simulink model "L3G4200D_SPI_interface"  (R2015a)
settings: Solver=FixedStepDiscrete  SolverMode=SingleTasking  StartTime=0.0  StopTime=inf  FixedStep=.001  RelTol=1e-3
model workspace (MAT data in the model file):
  message_length = Simulink.Parameter
  message_length.Value = 16
  message_length.DataType = 'uint16'
  clk_freq = Simulink.Parameter
  clk_freq.Value = 1000000
  clk_freq.DataType = 'uint32'
  cs_to_clk_edge = Simulink.Parameter
  cs_to_clk_edge.Value = 10
  cs_to_clk_edge.DataType = 'uint16'
  stall_time = Simulink.Parameter
  stall_time.Value = 4
  stall_time.DataType = 'uint16'
  Tcount_max = 20
  Tstall_max = 2000
  PAGE_0 = 32768
  PAGE_1 = 32769
  PAGE_2 = 32770
  PAGE_3 = 32771
  DEC_RATE_984a = 35864
  DEC_RATE_984b = 36096
  Z_ACCL_OUT = 9728
  PROD_ID = 32256
  CTRL_REG1_L3G = 8399
  OUT_X_L_L3G = 43008
  OUT_X_H_L3G = 43264
  OUT_Y_L_L3G = 43520
  OUT_Y_H_L3G = 43776
  OUT_Z_L_L3G = 44032
  OUT_Z_H_L3G = 44288
  read_table_L3G = [43008 43264 43520 43776 44032 44288 36608]
  WHO_AM_I_L3G = 36608
  init_cmd_L3G = 8399
undefined symbols (not defined in the file): AXI4, Lite
libraries: axiinterfacelib x8
settings Model: FPTRunName=FPA_Reference  SimulationMode=external  RecordCoverage=on  CovPath=/hdl_dut/Transmit  CovMetricSettings=r  CovHtmlReporting=off  CovReportOnPause=off  CovSFcnEnable=off  Creator=dlwalter  LastModifiedBy=dlwalter
settings OptimizationCC: BlockReduction=off  BooleanDataType=off  ConditionallyExecuteInputs=off  OptimizeModelRefInitCode=on  LifeSpan=2  MaxStackSize=64
settings DebuggingCC: AlgebraicLoopMsg=error  SaveWithParameterizedLinksMsg=none  UnderspecifiedInitializationDetection=Classic  MergeDetectMultiDrivingBlocksExec=none  SignalResolutionControl=TryResolveAllWithWarning
settings HardwareCC: ProdLargestAtomicInteger=Long  ProdLargestAtomicFloat=Double  ProdEndianess=LittleEndian  ProdHWDeviceType=ARM Compatible->ARM Cortex  TargetUnknown=on  ProdEqTarget=off
settings RTWCC: SystemTargetFile=ert.tlc  TLCOptions=-aInlineSetEventsForThisBaseRateFcn=TLC_FALSE -aSuppressMultiTaskScheduler=TLC_FALSE  TemplateMakefile=ert_default_tmf  Description=Embedded Coder  Toolchain=Xilinx Software Development Kit (SDK) 2013.4
settings CodeAppCC: IgnoreCustomStorageClasses=off
settings ERTTargetCC: GenerateSampleERTMain=off  ParMdlRefBuildCompliant=on  CompOptLevelCompliant=on  ConcurrentExecutionCompliant=on  ERTFirstTimeCompliant=on  SupportContinuousTime=off  SupportVariableSizeSignals=off  ModelStepFunctionPrototypeControlCompliant=on  CPPClassGenCompliant=on

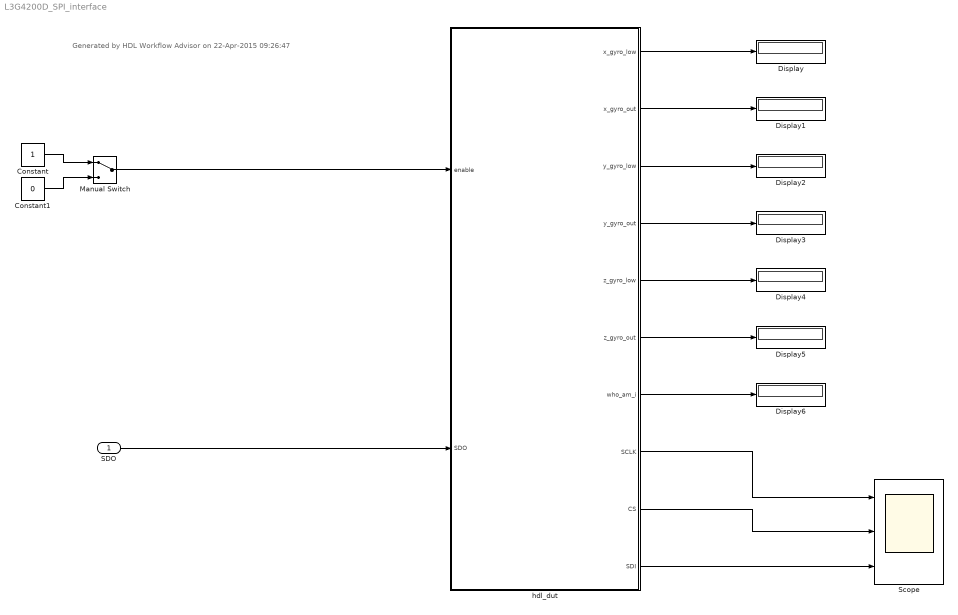
== system L3G4200D_SPI_interface ==
  note: Generated by HDL Workflow Advisor on 22-Apr-2015 09:26:47
  SDO : Inport
  Constant : Constant  OutDataTypeStr=boolean  SampleTime=-1
  Constant1 : Constant  Value=0  OutDataTypeStr=boolean  SampleTime=-1
  Display{,1..6} (7 alike) : Display
      Display6 settings: Format=octal (Stored Integer)
  Manual Switch : ManualSwitch
  Scope : Scope  NumInputPorts=3
      settings: TimeRange=3000  YMin=-5~-5~-5  YMax=5~5~5
  hdl_dut : Subsystem  TreatAsAtomicUnit=on  MinMaxOverflowLogging=MinMaxAndOverflow  mask(AXI4-Lite/AXI4 Interface){}
      mask help:
      | This is an automatically generated subsystem block.
      | This contains the AXI4-Lite/AXI4 interface which communicates with the L3G4200D_SPI_hdl_dut_ipcore IPCore generated from L3G4200D_SPI/hdl_dut subsystem.
      mask Display: disp(sprintf('Xilinx Zynq \nAXI4-Lite/AXI4 Interface'));
  wires:
  Constant1/1 -> Manual Switch/2
  Constant/1 -> Manual Switch/1
  hdl_dut/10(SDI) -> Scope/3
  hdl_dut/9(CS) -> Scope/2
  hdl_dut/8(SCLK) -> Scope/1
  hdl_dut/7(who_am_i) -> Display6/1
  hdl_dut/5(z_gyro_low) -> Display4/1
  hdl_dut/6(z_gyro_out) -> Display5/1
  hdl_dut/4(y_gyro_out) -> Display3/1
  hdl_dut/3(y_gyro_low) -> Display2/1
  hdl_dut/2(x_gyro_out) -> Display1/1
  hdl_dut/1(x_gyro_low) -> Display/1
  SDO/1 -> hdl_dut/2(SDO)
  Manual Switch/1 -> hdl_dut/1(enable)

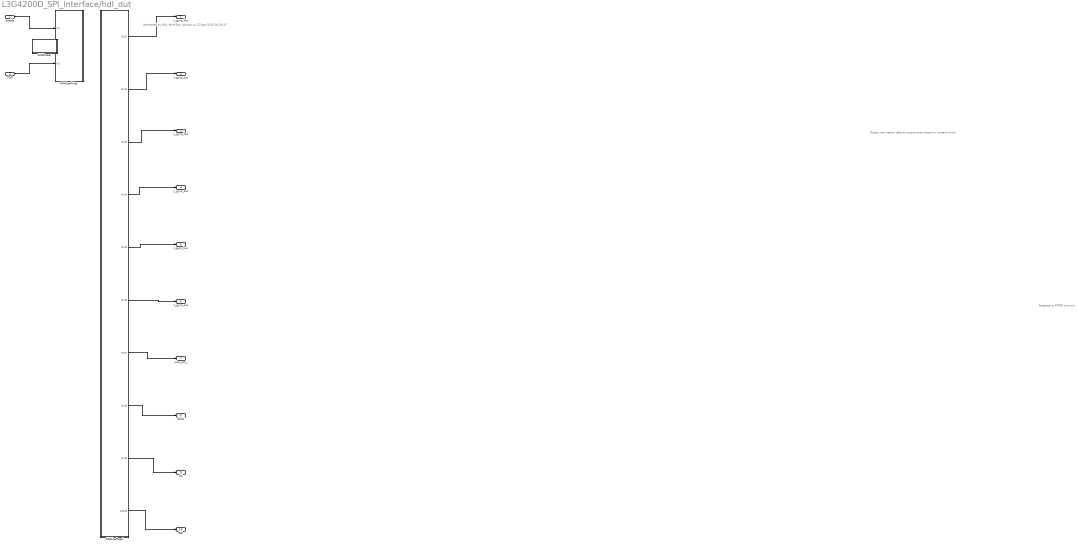
== system L3G4200D_SPI_interface/hdl_dut ==
  note: Assigned to PMOD pins out
  note: Assign new sensor data to output array based on current count
  note: Generated by HDL Workflow Advisor on 22-Apr-2015 09:26:47
  enable : Inport
  SDO : Inport  Port=2
  AXI4LiteRead : Subsystem  Priority=10
  AXI4LiteWrite : Subsystem  Priority=1
  AXI4Reset : Subsystem  mask(System Initialize){ShowInLibBrowser=0}
      mask prompts: ShowInLibBrowser "Simulink:masks:CustCodeMaskParam1_MP"
      settings: CopyFcn=cccopyfcn(gcb)  OpenFcn=ccopenfcn('System Initialize Function')
      mask Help: eval('feval(''rtwprivate'',''rtwhelpview'',''rtw_sys_initialize_block'')');
      mask Display: disp('System\nInitialize');
  x_gyro_low : Outport
  x_gyro_out : Outport  Port=2
  y_gyro_low : Outport  Port=3
  y_gyro_out : Outport  Port=4
  z_gyro_low : Outport  Port=5
  z_gyro_out : Outport  Port=6
  who_am_i : Outport  Port=7
  SCLK : Outport  Port=8
  CS : Outport  Port=9
  SDI : Outport  Port=10
  wires:
  enable/1 -> AXI4LiteWrite/1(In1)
  SDO/1 -> AXI4LiteWrite/2(In2)
  AXI4LiteRead/1(Out1) -> x_gyro_low/1
  AXI4LiteRead/2(Out2) -> x_gyro_out/1
  AXI4LiteRead/3(Out3) -> y_gyro_low/1
  AXI4LiteRead/4(Out4) -> y_gyro_out/1
  AXI4LiteRead/5(Out5) -> z_gyro_low/1
  AXI4LiteRead/6(Out6) -> z_gyro_out/1
  AXI4LiteRead/7(Out7) -> who_am_i/1
  AXI4LiteRead/8(Out8) -> SCLK/1
  AXI4LiteRead/9(Out9) -> CS/1
  AXI4LiteRead/10(Out10) -> SDI/1

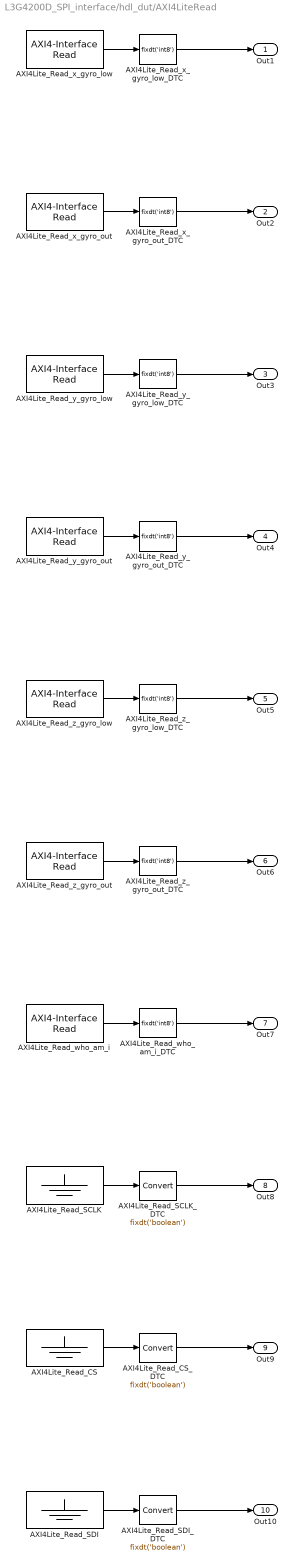
== system L3G4200D_SPI_interface/hdl_dut/AXI4LiteRead ==
  AXI4Lite_Read_CS : Ground
  AXI4Lite_Read_CS_DTC : DataTypeConversion  OutDataTypeStr=fixdt('boolean')  ConvertRealWorld=Stored Integer (SI)
  AXI4Lite_Read_SCLK : Ground
  AXI4Lite_Read_SCLK_DTC : DataTypeConversion  OutDataTypeStr=fixdt('boolean')  ConvertRealWorld=Stored Integer (SI)
  AXI4Lite_Read_SDI : Ground
  AXI4Lite_Read_SDI_DTC : DataTypeConversion  OutDataTypeStr=fixdt('boolean')  ConvertRealWorld=Stored Integer (SI)
  AXI4Lite_Read_who_am_i : axiinterfacelib/AXI4-Interface Read  Priority=8  AXIInterfaceType=AXI4-Lite  DeviceName=/dev/mwipcore  RegisterOffset=hex2dec('11C')  DataLength=4096  DataType=uint32  SampleTime=-1  blockPlatform=ZYNQ  SimulateUsing=Interpreted Execution
  AXI4Lite_Read_who_am_i_DTC : DataTypeConversion  OutDataTypeStr=fixdt('int8')  ConvertRealWorld=Stored Integer (SI)
  AXI4Lite_Read_x_gyro_low : axiinterfacelib/AXI4-Interface Read  Priority=2  AXIInterfaceType=AXI4-Lite  DeviceName=/dev/mwipcore  RegisterOffset=hex2dec('104')  DataLength=4096  DataType=uint32  SampleTime=-1  blockPlatform=ZYNQ  SimulateUsing=Interpreted Execution
  AXI4Lite_Read_x_gyro_low_DTC : DataTypeConversion  OutDataTypeStr=fixdt('int8')  ConvertRealWorld=Stored Integer (SI)
  AXI4Lite_Read_x_gyro_out : axiinterfacelib/AXI4-Interface Read  Priority=3  AXIInterfaceType=AXI4-Lite  DeviceName=/dev/mwipcore  RegisterOffset=hex2dec('108')  DataLength=4096  DataType=uint32  SampleTime=-1  blockPlatform=ZYNQ  SimulateUsing=Interpreted Execution
  AXI4Lite_Read_x_gyro_out_DTC : DataTypeConversion  OutDataTypeStr=fixdt('int8')  ConvertRealWorld=Stored Integer (SI)
  AXI4Lite_Read_y_gyro_low : axiinterfacelib/AXI4-Interface Read  Priority=4  AXIInterfaceType=AXI4-Lite  DeviceName=/dev/mwipcore  RegisterOffset=hex2dec('10C')  DataLength=4096  DataType=uint32  SampleTime=-1  blockPlatform=ZYNQ  SimulateUsing=Interpreted Execution
  AXI4Lite_Read_y_gyro_low_DTC : DataTypeConversion  OutDataTypeStr=fixdt('int8')  ConvertRealWorld=Stored Integer (SI)
  AXI4Lite_Read_y_gyro_out : axiinterfacelib/AXI4-Interface Read  Priority=5  AXIInterfaceType=AXI4-Lite  DeviceName=/dev/mwipcore  RegisterOffset=hex2dec('110')  DataLength=4096  DataType=uint32  SampleTime=-1  blockPlatform=ZYNQ  SimulateUsing=Interpreted Execution
  AXI4Lite_Read_y_gyro_out_DTC : DataTypeConversion  OutDataTypeStr=fixdt('int8')  ConvertRealWorld=Stored Integer (SI)
  AXI4Lite_Read_z_gyro_low : axiinterfacelib/AXI4-Interface Read  Priority=6  AXIInterfaceType=AXI4-Lite  DeviceName=/dev/mwipcore  RegisterOffset=hex2dec('114')  DataLength=4096  DataType=uint32  SampleTime=-1  blockPlatform=ZYNQ  SimulateUsing=Interpreted Execution
  AXI4Lite_Read_z_gyro_low_DTC : DataTypeConversion  OutDataTypeStr=fixdt('int8')  ConvertRealWorld=Stored Integer (SI)
  AXI4Lite_Read_z_gyro_out : axiinterfacelib/AXI4-Interface Read  Priority=7  AXIInterfaceType=AXI4-Lite  DeviceName=/dev/mwipcore  RegisterOffset=hex2dec('118')  DataLength=4096  DataType=uint32  SampleTime=-1  blockPlatform=ZYNQ  SimulateUsing=Interpreted Execution
  AXI4Lite_Read_z_gyro_out_DTC : DataTypeConversion  OutDataTypeStr=fixdt('int8')  ConvertRealWorld=Stored Integer (SI)
  Out1 : Outport
  Out2 : Outport  Port=2
  Out3 : Outport  Port=3
  Out4 : Outport  Port=4
  Out5 : Outport  Port=5
  Out6 : Outport  Port=6
  Out7 : Outport  Port=7
  Out8 : Outport  Port=8
  Out9 : Outport  Port=9
  Out10 : Outport  Port=10
  wires:
  AXI4Lite_Read_x_gyro_low/1 -> AXI4Lite_Read_x_gyro_low_DTC/1
  AXI4Lite_Read_x_gyro_low_DTC/1 -> Out1/1
  AXI4Lite_Read_y_gyro_low/1 -> AXI4Lite_Read_y_gyro_low_DTC/1
  AXI4Lite_Read_x_gyro_out_DTC/1 -> Out2/1
  AXI4Lite_Read_x_gyro_out/1 -> AXI4Lite_Read_x_gyro_out_DTC/1
  AXI4Lite_Read_y_gyro_out_DTC/1 -> Out4/1
  AXI4Lite_Read_y_gyro_low_DTC/1 -> Out3/1
  AXI4Lite_Read_y_gyro_out/1 -> AXI4Lite_Read_y_gyro_out_DTC/1
  AXI4Lite_Read_z_gyro_low/1 -> AXI4Lite_Read_z_gyro_low_DTC/1
  AXI4Lite_Read_z_gyro_out/1 -> AXI4Lite_Read_z_gyro_out_DTC/1
  AXI4Lite_Read_z_gyro_out_DTC/1 -> Out6/1
  AXI4Lite_Read_z_gyro_low_DTC/1 -> Out5/1
  AXI4Lite_Read_SCLK/1 -> AXI4Lite_Read_SCLK_DTC/1
  AXI4Lite_Read_who_am_i_DTC/1 -> Out7/1
  AXI4Lite_Read_CS/1 -> AXI4Lite_Read_CS_DTC/1
  AXI4Lite_Read_CS_DTC/1 -> Out9/1
  AXI4Lite_Read_SCLK_DTC/1 -> Out8/1
  AXI4Lite_Read_who_am_i/1 -> AXI4Lite_Read_who_am_i_DTC/1
  AXI4Lite_Read_SDI/1 -> AXI4Lite_Read_SDI_DTC/1
  AXI4Lite_Read_SDI_DTC/1 -> Out10/1

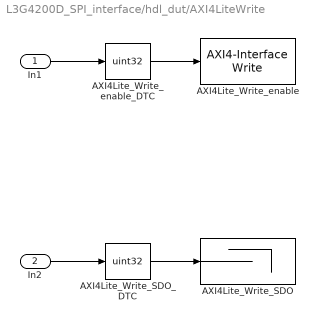
== system L3G4200D_SPI_interface/hdl_dut/AXI4LiteWrite ==
  In1 : Inport
  In2 : Inport  Port=2
  AXI4Lite_Write_SDO : Terminator
  AXI4Lite_Write_SDO_DTC : DataTypeConversion  OutDataTypeStr=uint32  ConvertRealWorld=Stored Integer (SI)
  AXI4Lite_Write_enable : axiinterfacelib/AXI4-Interface Write  Priority=1  AXIInterfaceType=AXI4-Lite  DeviceName=/dev/mwipcore  RegisterOffset=hex2dec('100')  blockPlatform=ZYNQ  SimulateUsing=Interpreted execution
  AXI4Lite_Write_enable_DTC : DataTypeConversion  OutDataTypeStr=uint32  ConvertRealWorld=Stored Integer (SI)
  wires:
  In1/1 -> AXI4Lite_Write_enable_DTC/1
  AXI4Lite_Write_SDO_DTC/1 -> AXI4Lite_Write_SDO/1
  In2/1 -> AXI4Lite_Write_SDO_DTC/1
  AXI4Lite_Write_enable_DTC/1 -> AXI4Lite_Write_enable/1

== system L3G4200D_SPI_interface/hdl_dut/AXI4Reset ==
